simulink model "CALC"  (R2021a)
settings: Solver=VariableStepAuto  StartTime=0.0  StopTime=10.0  RelTol=1e-3
settings Model: Creator=Osman  LastModifiedBy=Osman

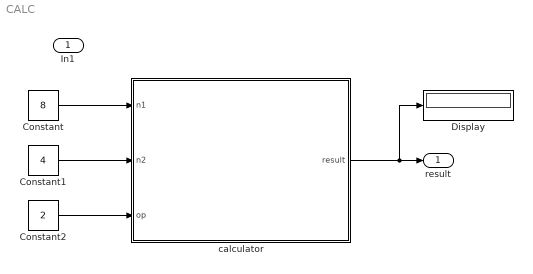
== system CALC ==
  In1 : Inport
  Constant : Constant  Value=8  OutDataTypeStr=int64
  Constant1 : Constant  Value=4  OutDataTypeStr=int64
  Constant2 : Constant  Value=2  OutDataTypeStr=uint8
  Display : Display
  calculator : Stateflow chart  TreatAsAtomicUnit=on
  result : Outport
  wires:
  calculator/1(result) -> Display/1, result/1
  Constant/1 -> calculator/1(n1)
  Constant1/1 -> calculator/2(n2)
  Constant2/1 -> calculator/3(op)

== stateflow chart CALC/calculator ==
  state add(num1,num2) [function]
    (default) -> (junction 39) : {result = (num1+num2);}
  state sub(num1, num2) [function]
    (default) -> (junction 42) : {result = num1 - num2;}
  state mult(num1,num2) [function]
    (default) -> (junction 46) : {result = num1 * num2;}
  state div(num1,num2) [function]
    (default) -> (junction 47)
    (junction 47) -> (junction 58) [order 1] : [num2 == 0]
    (junction 47) -> (junction 59) [order 2] : {result = num1/num2;}
    (junction 58) -> (junction 62) : {result = -1;}
    (junction 62) -> (junction 59)
  (default) -> (junction 16) : % calculator
  (junction 16) -> (junction 17) [order 1] : [op == 0]
  (junction 16) -> (junction 18) [order 2]
  (junction 17) -> (junction 25) : {add(n1,n2);}
  (junction 18) -> (junction 19) [order 1] : [op == 1]
  (junction 18) -> (junction 20) [order 2]
  (junction 19) -> (junction 24) : {sub(n1,n2);}
  (junction 20) -> (junction 21) [order 1] : [op == 2]
  (junction 20) -> (junction 22) [order 2]
  (junction 21) -> (junction 23) : {mult(n1,n2);}
  (junction 22) -> (junction 27) [order 1] : [op == 3]
  (junction 22) -> (junction 32) [order 2]
  (junction 27) -> (junction 29) : {div(n1,n2);}
  (junction 29) -> (junction 32)
  (junction 23) -> (junction 29)
  (junction 24) -> (junction 23)
  (junction 25) -> (junction 24)
  (junction 32) -> (junction 35)
  data: num1 function_input; num2 function_input; num1 function_input; num2 function_input; num1 function_input; num2 function_input; num1 function_input; num2 function_input; n1 input int64; n2 input int64; op input uint8; result output int64
